simulink model "Grid_control_using_PQ"  (R2019b)
settings: Solver=VariableStepAuto  StartTime=0.0  StopTime=10.0  RelTol=1e-3
libraries: powerlib x13, powerlib_meascontrol x4
settings Model: Creator=shiva  LastModifiedBy=shiva

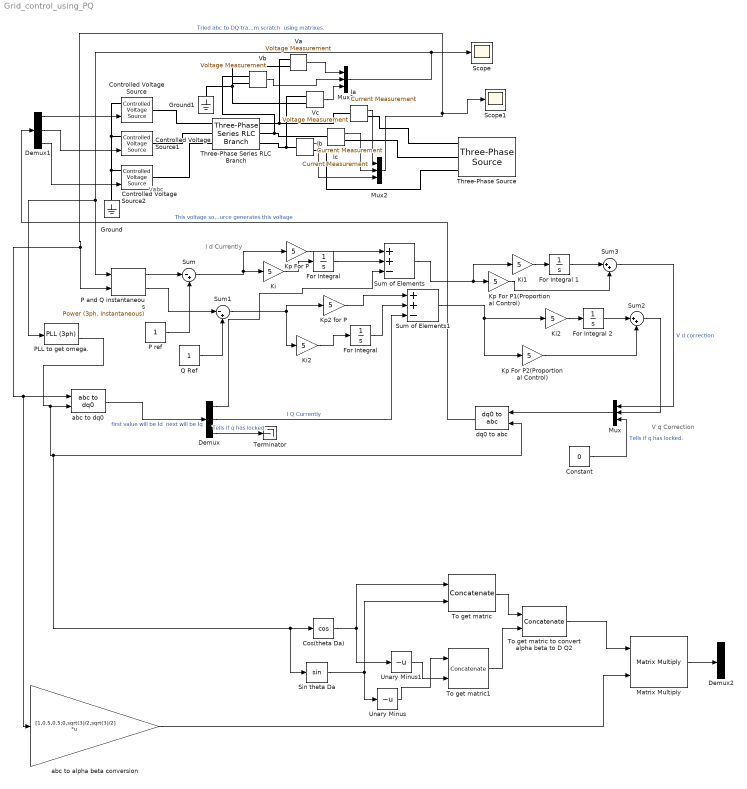
== system Grid_control_using_PQ ==
  note: V q Correction
  note: I d Currently
  note: Vabc
  Constant : Constant  Value=0
  Controlled Voltage Source : powerlib/Electrical Sources/Controlled Voltage Source  Initialize=on  Source_Type=AC  Amplitude=220  Phase=0  Frequency=0  Measurements=Voltage
      settings: SourceProductName=Simscape Electrical
  Controlled Voltage Source1 : powerlib/Electrical Sources/Controlled Voltage Source  Initialize=on  Source_Type=AC  Amplitude=220  Phase=0  Frequency=0  Measurements=None
      settings: SourceProductName=Simscape Electrical
  Controlled Voltage Source2 : powerlib/Electrical Sources/Controlled Voltage Source  Initialize=on  Source_Type=AC  Amplitude=220  Phase=0  Frequency=0  Measurements=None
      settings: SourceProductName=Simscape Electrical
  Cos(theta Da) : Trigonometry  Operator=cos
  Demux : Demux  Outputs=3
  Demux1 : Demux  Outputs=3
  Demux2 : Demux  Outputs=2
  For Integral : Integrator
  "For Integral " : Integrator
  For Integral 1 : Integrator
  For Integral 2 : Integrator
  Ground : powerlib/Elements/Ground  LConnTagsString=a
      settings: SourceProductName=Simscape Electrical
  Ground1 : powerlib/Elements/Ground  LConnTagsString=a
      settings: SourceProductName=Simscape Electrical
  Ia : powerlib/Measurements/Current Measurement  PhasorSimulation=off  OutputType=Complex  PSBequivalent=0
      settings: SourceProductName=Simscape Electrical
  Ib : powerlib/Measurements/Current Measurement  PhasorSimulation=off  OutputType=Complex  PSBequivalent=0
      settings: SourceProductName=Simscape Electrical
  Ic : powerlib/Measurements/Current Measurement  PhasorSimulation=off  OutputType=Complex  PSBequivalent=0
      settings: SourceProductName=Simscape Electrical
  Ki : Gain  Gain=5
  Ki1 : Gain  Gain=5
  Ki2 : Gain  Gain=5
  "Ki2 " : Gain  Gain=5
  Kp For P : Gain  Gain=5
  Kp For P1(Proportional Control) : Gain  Gain=5
  Kp For P2(Proportional Control) : Gain  Gain=5
  Kp2 for P : Gain  Gain=5
  Matrix Multiply : Product  Multiplication=Matrix(*)
  Mux : Mux  Inputs=3
  Mux1 : Mux  Inputs=3
  Mux2 : Mux  Inputs=3
  P and Q instantaneous : powerlib_meascontrol/Measurements/Power (3ph, Instantaneous)
      settings: SourceProductName=Simscape Electrical
  "P ref " : Constant
  "PLL to get omega. " : powerlib_meascontrol/PLL/PLL (3ph)  Fmin=45  Par_Init=[0, 50]  ParK=[180, 3200, 1]  TcD=1e-4  MaxRateChangeFreq=12  FilterCutOffFreq=25  Ts=0  AGC=on
      settings: SourceProductName=Simscape Electrical
  "Q Ref " : Constant
  Scope : Scope
  Scope1 : Scope
  Sin theta Da : Trigonometry
  Sum : Sum  Inputs=|-+
  Sum of Elements : Sum  Inputs=++-
  Sum of Elements1 : Sum  Inputs=++-
  Sum1 : Sum  Inputs=|-+
  Sum2 : Sum  Inputs=|++
  Sum3 : Sum  Inputs=|++
  Terminator : Terminator
  Three-Phase Series RLC Branch : powerlib/Elements/Three-Phase Series RLC Branch  LConnTagsString=A|B|C  RConnTagsString=A|B|C  BranchType=L  Resistance=1  Inductance=1e-3  Capacitance=1e-6  Measurements=None
      settings: SourceProductName=Simscape Electrical
  Three-Phase Source : powerlib/Electrical Sources/Three-Phase Source  InternalConnection=Y  VoltagePhases=on  Voltage=25e3  PhaseAngle=0  Voltage_phases=[220 220 220]  PhaseAngles_phases=[0 -120 +120]  Frequency=50  NonIdealSource=on  SpecifyImpedance=off  Resistance=.0001  Inductance=16.58e-6  ShortCircuitLevel=100e6  BaseVoltage=220  XRratio=7  BusType=swing  Pref=10e3  Qref=0  Prefabc=[10e3, 10e3, 10e3]  Qrefabc=[0, 0, 0]  Qmin=-inf  Qmax=inf
      settings: SourceProductName=Simscape Electrical
  "To get matric " : Concatenate
  To get matric to convert alpha beta to D Q2 : Concatenate  Mode=Multidimensional array  ConcatenateDimension=2
  To get matric1 : Concatenate
  Unary Minus : UnaryMinus
  Unary Minus1 : UnaryMinus
  Va : powerlib/Measurements/Voltage Measurement  PhasorSimulation=off  OutputType=Complex  PSBequivalent=0
      settings: SourceProductName=Simscape Electrical
  Vb : powerlib/Measurements/Voltage Measurement  PhasorSimulation=off  OutputType=Complex  PSBequivalent=0
      settings: SourceProductName=Simscape Electrical
  Vc : powerlib/Measurements/Voltage Measurement  PhasorSimulation=off  OutputType=Complex  PSBequivalent=0
      settings: SourceProductName=Simscape Electrical
  "abc to alpha beta conversion " : Gain  Gain=[1,0.5,0.5;0,sqrt(3)/2,sqrt(3)/2]  Multiplication=Matrix(K*u)
  abc to dq0 : powerlib_meascontrol/Transformations/abc to dq0  Alignment=90 degrees behind phase A axis
      settings: SourceProductName=Simscape Electrical
  dq0 to abc : powerlib_meascontrol/Transformations/dq0 to abc  Alignment=90 degrees behind phase A axis
      settings: SourceProductName=Simscape Electrical
  wires:
  Mux1/1 -> P and Q instantaneous/1, "PLL to get omega. "/1, Scope/1
  P and Q instantaneous/1 -> Sum/1
  "P ref "/1 -> Sum/2
  P and Q instantaneous/2 -> Sum1/1
  "Q Ref "/1 -> Sum1/2
  Sum/1 -> Ki/1, Kp For P/1
  Ki/1 -> "For Integral "/1
  For Integral/1 -> Sum of Elements1/2
  "Ki2 "/1 -> For Integral/1
  Sum1/1 -> "Ki2 "/1, Kp2 for P/1
  abc to dq0/1 -> Demux/1  "first value will be Id  next will be Iq"
  Demux/2 -> Sum of Elements1/3  "I Q Currently"
  "For Integral "/1 -> Sum of Elements/2
  Demux/1 -> Sum of Elements/3
  Ki1/1 -> For Integral 1/1
  For Integral 1/1 -> Sum3/1
  Sum of Elements/1 -> Ki1/1, Kp For P1(Proportional Control)/1
  For Integral 2/1 -> Sum2/1
  Ki2/1 -> For Integral 2/1
  Sum of Elements1/1 -> Ki2/1, Kp For P2(Proportional Control)/1
  Sum3/1 -> Mux/1  "V d correction"
  Sum2/1 -> Mux/2
  Mux/1 -> dq0 to abc/1
  dq0 to abc/1 -> Demux1/1  "This voltage source generates this voltage"
  Constant/1 -> Mux/3  "Tells if q has locked."
  Demux1/1 -> Controlled Voltage Source/1
  Demux1/2 -> Controlled Voltage Source1/1
  Demux1/3 -> Controlled Voltage Source2/1
  Ia/1 -> Mux2/1
  Ic/1 -> Mux2/2
  Ib/1 -> Mux2/3
  Va/1 -> Mux1/1
  Vb/1 -> Mux1/2
  Vc/1 -> Mux1/3
  Unary Minus1/1 -> To get matric1/2
  "To get matric "/1 -> To get matric to convert alpha beta to D Q2/1
  Matrix Multiply/1 -> Demux2/1
  Sin theta Da/1 -> Unary Minus/1, "To get matric "/2
  Cos(theta Da)/1 -> "To get matric "/1, Unary Minus1/1
  Mux2/1 -> Scope1/1, P and Q instantaneous/2, "abc to alpha beta conversion "/1, abc to dq0/1  "Tried abc to DQ transformation  from scratch  using matrixes."
  "PLL to get omega. "/2 -> abc to dq0/2, Sin theta Da/1, Cos(theta Da)/1, dq0 to abc/2
  To get matric to convert alpha beta to D Q2/1 -> Matrix Multiply/1
  "abc to alpha beta conversion "/1 -> Matrix Multiply/2
  To get matric1/1 -> To get matric to convert alpha beta to D Q2/2
  Unary Minus/1 -> To get matric1/1
  Demux/3 -> Terminator/1  "Tells if q has locked."
  Kp For P/1 -> Sum of Elements/1
  Kp2 for P/1 -> Sum of Elements1/1
  Kp For P1(Proportional Control)/1 -> Sum3/2
  Kp For P2(Proportional Control)/1 -> Sum2/2
  connections:
  Ground/LConn1 -- Controlled Voltage Source2/LConn1 -- Controlled Voltage Source1/LConn1 -- Controlled Voltage Source/LConn1
  Controlled Voltage Source/RConn1 -- Three-Phase Series RLC Branch/LConn1
  Controlled Voltage Source1/RConn1 -- Three-Phase Series RLC Branch/LConn2
  Controlled Voltage Source2/RConn1 -- Three-Phase Series RLC Branch/LConn3
  Ia/LConn1 -- Va/LConn1 -- Three-Phase Series RLC Branch/RConn1
  Three-Phase Series RLC Branch/RConn2 -- Vb/LConn1 -- Ic/LConn1
  Three-Phase Series RLC Branch/RConn3 -- Vc/LConn1 -- Ib/LConn1
  Three-Phase Source/RConn1 -- Ia/RConn1
  Three-Phase Source/RConn2 -- Ic/RConn1
  Three-Phase Source/RConn3 -- Ib/RConn1
  Ground1/LConn1 -- Va/LConn2 -- Vb/LConn2 -- Vc/LConn2
